simulink model "PR_Planar_Testbench_2018"  (R2024a)
settings: Solver=FixedStepDiscrete  StartTime=0.0  StopTime=inf  FixedStep=param.t_sample  RelTol=1e-3
undefined symbols (not defined in the file): max_qa, min_qa, param, slave3
libraries: Cust_Library_planarPKM x54, simulink_extras x27, dspswit3 x24, simulink x22, etherlab_lib x12
(part 2 of 6)

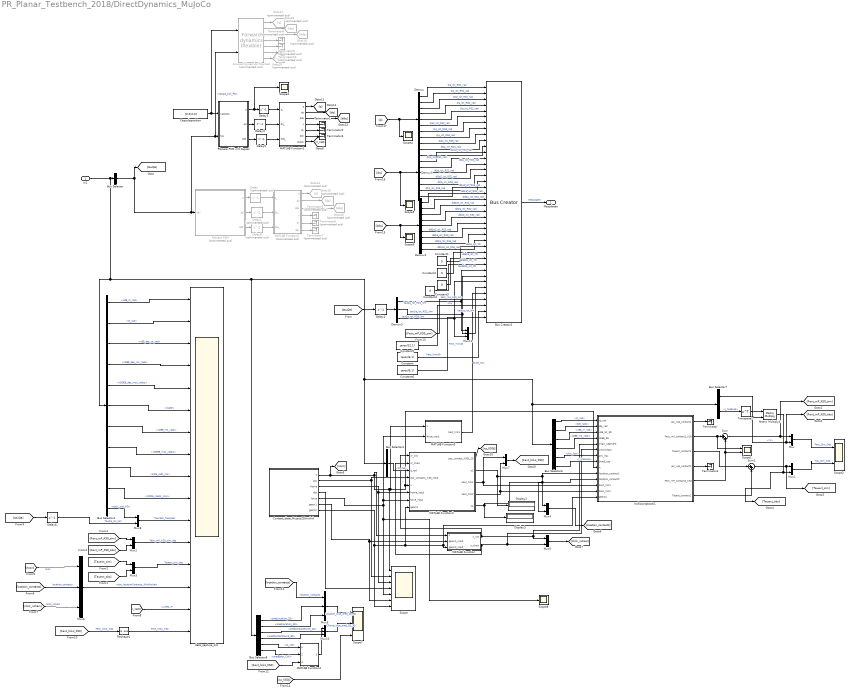
== system PR_Planar_Testbench_2018/DirectDynamics_MuJoCo ==
  In1 : Inport
  Bus Creator2 : BusCreator  Inputs=40
  Bus Selector : BusSelector  OutputSignals=PD_Controller.TauQa_soll_PD
  Bus Selector1 : BusSelector  OutputSignals=Kinematics_currentValues.xEE_m_rad,Kinematics_currentValues.Q_rad,Logical data.xEE_des_m_rad,Logical data.xDEE_des_ms_rads,Logical data.xDDEE_des_mss_radss,Logical data.state,Differential kinematics - current values.xDEE_ms_rads,Differential kinematics - current values.xDDEE_mss_radss,Differential kinematics - current values.QDa_rads_ms,Differential kinematics - current values.QDDa_radss_mss,PD_Controller.tauX_soll_PD
  Bus Selector4 : BusSelector  OutputSignals=Kinematics_currentValues.Q_rad
  Bus Selector6 : BusSelector  OutputSignals=Kinematics_currentValues.Q_rad,Differential kinematics - current values.QD_rads,Kinematics_currentValues.xEE_m_rad,Differential kinematics - current values.xDEE_ms_rads,Differential kinematics - current values.Jinv_hqx,Differential kinematics - current values.J_hredxqa
  Bus Selector7 : BusSelector  OutputSignals=Beobachter.rx,Differential kinematics - current values.J_hredxqa
  Bus Selector8 : BusSelector  OutputSignals=Beobachter.predLocation_2D,Beobachter.predLocation_3D,Beobachter.predContactForce_2D,Beobachter.predContactForce_3D,Kinematics_currentValues.Q_rad,Beobachter.predBody_Coll
  Capsuleposition : Constant  Value=[0;0;0;0]  SampleTime=-1
  Constant : Constant  Value=zeros(6,1)  SampleTime=-1
  Constant{1..4} (4 alike) : Constant  Value=0  SampleTime=-1
  Constant5 : Constant  Value=zeros(12,1)  SampleTime=-1
  Constant6 : Constant  Value=zeros(6,1)  SampleTime=-1
  Contact_data_Mujoco2Simulink : MATLAB Function  TreatAsAtomicUnit=on
  Delay : Delay  Commented=on  DelayLength=1  InitialCondition=param.q0_mj
  Delay1 : Delay  Commented=on  DelayLength=1
  Delay{2,4..6} (4 alike) : Delay  DelayLength=1
  Delay3 : Delay  DelayLength=1  InitialCondition=param.q0_mj
  Delay8 : Delay  Commented=on  DelayLength=1
  Demux : Demux  Outputs=9
  Demux1 : Demux  Outputs=9
  Demux2 : Demux  Outputs=9
  Demux3 : Demux  Outputs=3
  Display2 : Display
  Display3 : Display
  Forward dynamics (flexible) : Cust_Library_planarPKM/Forward dynamics (flexible)  Commented=on  capsule_active=param.capsule_active  t_sample=param.t_sample
  Goto14 : Goto  Commented=on  GotoTag=q
  Goto15 : Goto  Commented=on  GotoTag=dq
  Goto16 : Goto  Commented=on  GotoTag=ddq
  Goto17 : Goto  Commented=on  GotoTag=q
  Goto18 : Goto  Commented=on  GotoTag=dq
  Goto19 : Goto  Commented=on  GotoTag=ddq
  Goto20 : Goto  Commented=on  GotoTag=x_caps
  KollisionsJacobi1 : MATLAB Function  TreatAsAtomicUnit=on
  MATLAB Function : MATLAB Function  TreatAsAtomicUnit=on
  MATLAB Function1 : MATLAB Function  TreatAsAtomicUnit=on
  MATLAB Function2 : MATLAB Function  Commented=on  TreatAsAtomicUnit=on
  MATLAB Function3 : MATLAB Function  TreatAsAtomicUnit=on
  MATLAB Function4 : MATLAB Function  TreatAsAtomicUnit=on
  MATLAB Function5 : MATLAB Function  TreatAsAtomicUnit=on
  Matrix Multiply4 : Product  Multiplication=Matrix(*)
  Mux{,1..5,7..8} (8 alike) : Mux  Inputs=2
  Mux{6,9..11} (4 alike) : Mux  Inputs=3
  Planare PKM : MATLAB Function  Commented=on  TreatAsAtomicUnit=on
  Planare PKM mit Kapsel : MATLAB Function  TreatAsAtomicUnit=on
  Reshape1 : Reshape
  Scope : Scope  NumInputPorts=7
  Scope1 : Scope  NumInputPorts=2
  Scope2 : Scope  NumInputPorts=2
  Scope{3..6,8} (5 alike) : Scope
  Scope7 : Scope  NumInputPorts=3
  Sum : Sum  Inputs=|++
  Sum1 : Sum  Inputs=|++
  Terminator{,1..4} (5 alike) : Terminator
  Terminator{5..10} (6 alike) : Terminator  Commented=on
  Transpose2 : Math  Operator=transpose  SignedPower=on
  data_capture_sim : Scope  NumInputPorts=16
  Messdaten : Outport
  wires:
  Demux/9 -> Bus Creator2/9  "Qp2_ist_RS3_rad"
  Demux1/3 -> Bus Creator2/12  "dQp2_ist_RS1_rad"
  Demux1/8 -> Bus Creator2/17  "dQp_ist_RS3_rad"
  Demux3/3 -> Bus Creator2/34, Mux11/3  "tauQa_ist_RD3_Nm"
  Demux1/1 -> Bus Creator2/10  "dQa_ist_RD1_rad"
  Demux/2 -> Bus Creator2/2  "Qp_ist_RS1_rad"
  Demux/1 -> Bus Creator2/1  "Qa_ist_RD1_rad"
  Demux/4 -> Bus Creator2/4  "Qa_ist_RD2_rad"
  Constant2/1 -> Bus Creator2/29  "ddelta_ist_TD"
  Bus Selector/1 -> [tauQa], Forward dynamics (flexible)/2, Planare PKM mit Kapsel/2(tau), Planare PKM/1(tau)  "<TauQa_soll_PD>"
  Demux/8 -> Bus Creator2/8  "Qp_ist_RS3_rad"
  Delay8/1 -> MATLAB Function2/3(ddq_)
  Demux3/2 -> Mux11/2, Bus Creator2/33  "tauQa_ist_RD2_Nm"
  MATLAB Function2/6(ddx) -> Terminator7/1
  Constant4/1 -> Bus Creator2/31  "taudelta_ist_TD"
  Demux/3 -> Bus Creator2/3  "Qp2_ist_RS1_rad"
  Demux1/7 -> Bus Creator2/16  "dQa_ist_RD3_rad"
  Demux2/5 -> Bus Creator2/23  "ddQp_ist_RS2_rad"
  Demux2/7 -> Bus Creator2/25  "ddQa_ist_RD3_rad"
  Delay2/1 -> Demux3/1
  Demux2/3 -> Bus Creator2/21  "ddQp2_ist_RS1_rad"
  Delay/1 -> MATLAB Function2/1(q_)
  Demux1/9 -> Bus Creator2/18  "dQp2_ist_RS3_rad"
  Demux2/8 -> Bus Creator2/26  "ddQp_ist_RS3_rad"
  Demux2/2 -> Bus Creator2/20  "ddQp_ist_RS1_rad"
  Demux2/4 -> Bus Creator2/22  "ddQa_ist_RD2_rad"
  Demux2/1 -> Bus Creator2/19  "ddQa_ist_RD1_rad"
  Demux1/5 -> Bus Creator2/14  "dQp_ist_RS2_rad"
  Planare PKM/1(q) -> Delay/1
  Demux2/6 -> Bus Creator2/24  "ddQp2_ist_RS2_rad"
  MATLAB Function2/5(dx) -> Terminator6/1
  Demux1/2 -> Bus Creator2/11  "dQp_ist_RS1_rad"
  Demux/5 -> Bus Creator2/5  "Qp_ist_RS2_rad"
  Demux1/4 -> Bus Creator2/13  "dQa_ist_RD2_rad"
  Planare PKM/2(qd) -> Delay1/1
  In1/1 -> Bus Selector8/1, Bus Selector4/1, Bus Selector7/1, Bus Selector6/1, Bus Selector1/1, Bus Selector/1
  Demux2/9 -> Bus Creator2/27  "ddQp2_ist_RS3_rad"
  Demux3/1 -> Mux11/1, Bus Creator2/32  "tauQa_ist_RD1_Nm"
  Constant1/1 -> Bus Creator2/28  "delta_ist_TD"
  Demux1/6 -> Bus Creator2/15  "dQp2_ist_RS2_rad"
  Demux/6 -> Bus Creator2/6  "Qp2_ist_RS2_rad"
  MATLAB Function2/4(x) -> Terminator5/1
  Planare PKM/3(qdd) -> Delay8/1
  Constant3/1 -> Bus Creator2/30  "dddelta_ist_TD"
  Delay1/1 -> MATLAB Function2/2(dq_)
  Demux/7 -> Bus Creator2/7  "Qa_ist_RD3_rad"
  [tauQa] -> Delay2/1
  Bus Creator2/1 -> Messdaten/1  "Messdaten"
  Planare PKM mit Kapsel/1(q) -> Scope3/1, Delay3/1
  Capsuleposition/1 -> Forward dynamics (flexible)/1, Planare PKM mit Kapsel/1(capspos)
  Planare PKM mit Kapsel/3(qdd) -> Delay5/1
  Delay3/1 -> MATLAB Function1/1(q_)
  Delay5/1 -> MATLAB Function1/3(ddq_)
  Delay4/1 -> MATLAB Function1/2(dq_)
  Planare PKM mit Kapsel/2(qd) -> Delay4/1
  MATLAB Function1/4(x) -> Terminator1/1
  MATLAB Function1/5(dx) -> Terminator2/1
  MATLAB Function1/6(ddx) -> Terminator3/1
  Contact_data_Mujoco2Simulink/7(geom2) -> MATLAB Function3/8(geom2), KollisionsJacobi1/14(geom2), MATLAB Function/3(geom2_input), Scope/7
  Contact_data_Mujoco2Simulink/5(force) -> MATLAB Function3/7(force_input), MATLAB Function5/2(force_input), Scope/5, Scope8/1
  Contact_data_Mujoco2Simulink/4(dist) -> Scope/4
  Contact_data_Mujoco2Simulink/3(frame) -> Scope/3, MATLAB Function3/6(frame_input)
  Contact_data_Mujoco2Simulink/2(pos) -> Scope/2, MATLAB Function3/4(pos_contacts_KS0_input)
  Contact_data_Mujoco2Simulink/1(n) -> [ncon], MATLAB Function/1(n), MATLAB Function5/1(n), MATLAB Function3/5(n), KollisionsJacobi1/9(n), Scope/1
  Contact_data_Mujoco2Simulink/6(geom1) -> Scope/6, MATLAB Function/2(geom1_input)
  Bus Selector1/1 -> data_capture_sim/1  "<xEE_m_rad>"
  Bus Selector1/2 -> data_capture_sim/2  "<Q_rad>"
  Bus Selector1/3 -> data_capture_sim/3  "<xEE_des_m_rad>"
  Bus Selector1/4 -> data_capture_sim/4  "<xDEE_des_ms_rads>"
  Bus Selector1/5 -> data_capture_sim/5  "<xDDEE_des_mss_radss>"
  Bus Selector1/6 -> data_capture_sim/6  "<state>"
  Bus Selector1/7 -> data_capture_sim/7  "<xDEE_ms_rads>"
  Bus Selector1/8 -> data_capture_sim/8  "<xDDEE_mss_radss>"
  Bus Selector1/9 -> data_capture_sim/9  "<QDa_rads_ms>"
  Bus Selector1/10 -> data_capture_sim/10  "<QDDa_radss_mss>"
  MATLAB Function3/3(Fext_link1) -> Mux7/1, KollisionsJacobi1/12(Fext_link1)
  MATLAB Function3/4(Fext_link2) -> Mux7/2, KollisionsJacobi1/13(Fext_link2)
  Bus Selector4/1 -> MATLAB Function3/3(q_rad)  "<Q_rad>"
  Bus Selector6/1 -> KollisionsJacobi1/1(qj_rad)  "<Q_rad>"
  Bus Selector6/2 -> KollisionsJacobi1/2(dqj_rad)  "<QD_rads>"
  Bus Selector6/3 -> KollisionsJacobi1/3(xEE_ist_3D)  "<xEE_m_rad>"
  Bus Selector6/4 -> KollisionsJacobi1/4(dxEE_3D)  "<xDEE_ms_rads>"
  Bus Selector6/5 -> KollisionsJacobi1/7(Jinv_hqx)  "<Jinv_hqx>"
  Bus Selector6/6 -> KollisionsJacobi1/8(Jhred_xqa)  "<J_hredxqa>"
  MATLAB Function3/2(s1) -> Display2/1, Mux4/1, KollisionsJacobi1/10(location_contact1)
  MATLAB Function3/5(s2) -> Mux4/2, KollisionsJacobi1/11(location_contact2), Display3/1
  KollisionsJacobi1/1(Jac_xpq_contact1) -> Terminator/1
  KollisionsJacobi1/4(Jac_xpq_contact2) -> Terminator4/1
  KollisionsJacobi1/2(Fext_mP_contact1_KS0) -> Scope1/1, Sum/1
  KollisionsJacobi1/5(Fext_mP_contact2_KS0) -> Scope1/2, Sum/2
  Sum1/1 -> [Tauext_sim], Mux1/1
  KollisionsJacobi1/3(Tauext_contact1) -> Sum1/1
  KollisionsJacobi1/6(Tauext_contact2) -> Sum1/2
  Bus Selector7/1 -> [Fext_mP_KS0_obs], Mux/2, Matrix Multiply4/2  "<rx>"
  Transpose2/1 -> Matrix Multiply4/1
  Bus Selector7/2 -> Transpose2/1  "<J_hredxqa>"
  Matrix Multiply4/1 -> Mux1/2, [Tauext_obs]
  Sum/1 -> [Fext_mP_KS0_sim], Mux/1
  Mux/1 -> Scope2/1  "Fext_Sim_Obs"
  Mux1/1 -> Scope2/2  "Tau_Sim_Obs"
  MATLAB Function/1(n_link) -> MATLAB Function3/1(nr_link), KollisionsJacobi1/5(chain_segment), Mux5/1
  MATLAB Function/2(n_chain) -> KollisionsJacobi1/6(whichchain), Mux5/2, MATLAB Function3/2(nr_chain)
  [Fext_mP_KS0_sim] -> Mux2/1
  [Fext_mP_KS0_obs] -> Mux2/2
  [Tauext_sim] -> Mux3/1
  [Tauext_obs] -> Mux3/2
  Mux2/1 -> data_capture_sim/12  "Fext_mP_KS0_sim_obs"
  Mux3/1 -> data_capture_sim/13  "Tauext_sim_obs"
  Mux4/1 -> [location_contacts]
  Mux5/1 -> [nlink_nchain]
  MATLAB Function1/7(qcaps) -> [x_caps]
  [ncon] -> Mux6/1  "ncon"
  [location_contacts] -> Mux6/2  "location_contacts"
  [nlink_nchain] -> Mux6/3  "nlink_nchain"
  Mux6/1 -> data_capture_sim/14  "ncon_locationContacts_NlinkNchain"
  [x_caps] -> data_capture_sim/15  "x_caps_m"
  [tauQa] -> Delay6/1
  Mux7/1 -> [Fext_links_KS0]
  [Fext_links_KS0] -> Reshape1/1  "Fext_links_KS0"
  Bus Selector1/11 -> Mux8/1  "<tauX_soll_PD>"
  Delay6/1 -> Mux8/2  "TauQa_ist_Nm"
  Mux8/1 -> data_capture_sim/11  "TauXSoll_TauQaIst"
  MATLAB Function1/1(q) -> [q]
  MATLAB Function1/2(dq) -> [dq]
  MATLAB Function1/3(ddq) -> [ddq]
  Bus Selector8/5 -> MATLAB Function4/1(q)  "<Q_rad>"
  Bus Selector8/6 -> MATLAB Function4/2(predBody)  "<predBody_Coll>"
  [Fext_links_KS0] -> MATLAB Function4/3(Fext_links_KS0)
  [location_contacts] -> Mux9/1  "location_contacts"
  Bus Selector8/1 -> Mux9/2  "<predLocation_2D>"
  Bus Selector8/3 -> Mux10/2  "<predContactForce_2D>"
  Mux9/1 -> Scope7/1  "Location_true_pred_2D_3D"
  Mux10/1 -> Scope7/2  "CForce_true_pred_2D_3D"
  MATLAB Function4/1(Fext_link_KSGj) -> Mux10/1
  Bus Selector8/4 -> Mux10/3  "<predContactForce_3D>"
  Bus Selector8/2 -> Mux9/3  "<predLocation_3D>"
  Mux11/1 -> Bus Creator2/35  "tauQa_ist_Nm"
  MATLAB Function5/1(Fext_link1) -> Bus Creator2/36  "force_mjc"
  [Fext_mP_KS0_sim] -> Bus Creator2/37  "Fext_mp_KS0_sim"
  MATLAB Function3/1(pos_contact_KSGj_2D) -> [xp_KSGj]
  [xp_KSGj] -> Scope7/3
  [q] -> Scope4/1, Demux/1
  [dq] -> Scope5/1, Demux1/1
  [ddq] -> Scope6/1, Demux2/1
  MATLAB Function2/2(dq) -> Goto15/1
  MATLAB Function2/3(ddq) -> Goto16/1
  MATLAB Function2/1(q) -> Goto14/1
  Constant5/1 -> Bus Creator2/38  "imu"
  Reshape1/1 -> data_capture_sim/16  "Fext_links_KS0"
  Constant6/1 -> Bus Creator2/40  "Fext_mini40"
  Constant/1 -> Bus Creator2/39  "Fext_kms40"
  Forward dynamics (flexible)/3 -> Goto19/1
  Forward dynamics (flexible)/2 -> Goto18/1
  Forward dynamics (flexible)/1 -> Goto17/1
  Forward dynamics (flexible)/7 -> Goto20/1
  Forward dynamics (flexible)/6 -> Terminator10/1
  Forward dynamics (flexible)/5 -> Terminator9/1
  Forward dynamics (flexible)/4 -> Terminator8/1

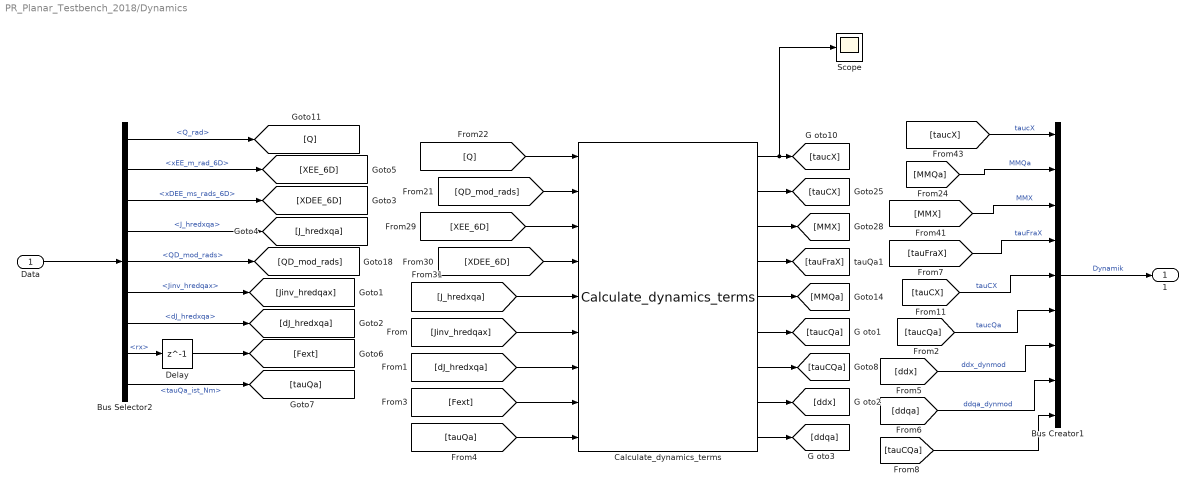
== system PR_Planar_Testbench_2018/Dynamics ==
  Data : Inport
  Bus Creator1 : BusCreator  Inputs=9
  Bus Selector2 : BusSelector  OutputSignals=Kinematics_currentValues.Q_rad,Kinematics_currentValues.xEE_m_rad_6D,Differential kinematics - current values.xDEE_ms_rads_6D,Differential kinematics - current values.J_hredxqa,Differential kinematics - current values.QD_mod_rads,Differential kinematics - current values.Jinv_hredqax,Differential kinematics - current values.dJ_hredxqa,Beobachter.rx,Messdaten.tauQa_ist_Nm
  Calculate_dynamics_terms : Cust_Library_planarPKM/Calculate_dynamics_terms  MDP=param.MDP  l_all=param.l_all  r_BasisPla_MobPla=param.r_BasisPla_MobPla
  Delay : Delay  DelayLength=1  InitialCondition=zeros(3,1)
  Scope : Scope
  1 : Outport
  wires:
  Bus Creator1/1 -> 1/1  "Dynamik"
  [taucX] -> Bus Creator1/1  "taucX"
  [MMX] -> Bus Creator1/3  "MMX"
  [tauFraX] -> Bus Creator1/4  "tauFraX"
  Bus Selector2/3 -> [XDEE_6D]  "<xDEE_ms_rads_6D>"
  Bus Selector2/1 -> [Q]  "<Q_rad>"
  Data/1 -> Bus Selector2/1
  Bus Selector2/4 -> [J_hredxqa]  "<J_hredxqa>"
  Bus Selector2/2 -> [XEE_6D]  "<xEE_m_rad_6D>"
  Bus Selector2/5 -> [QD_mod_rads]  "<QD_mod_rads>"
  [tauCX] -> Bus Creator1/5  "tauCX"
  [MMQa] -> Bus Creator1/2  "MMQa"
  [XEE_6D] -> Calculate_dynamics_terms/3
  [Q] -> Calculate_dynamics_terms/1
  [QD_mod_rads] -> Calculate_dynamics_terms/2
  [XDEE_6D] -> Calculate_dynamics_terms/4
  [J_hredxqa] -> Calculate_dynamics_terms/5
  Calculate_dynamics_terms/1 -> Scope/1, [taucX]
  Calculate_dynamics_terms/2 -> [tauCX]
  Calculate_dynamics_terms/3 -> [MMX]
  Calculate_dynamics_terms/4 -> [tauFraX]
  Calculate_dynamics_terms/5 -> [MMQa]
  Bus Selector2/6 -> [Jinv_hredqax]  "<Jinv_hredqax>"
  [Jinv_hredqax] -> Calculate_dynamics_terms/6
  Bus Selector2/7 -> [dJ_hredxqa]  "<dJ_hredxqa>"
  [dJ_hredxqa] -> Calculate_dynamics_terms/7
  Calculate_dynamics_terms/6 -> [taucQa]
  [taucQa] -> Bus Creator1/6  "taucQa"
  Bus Selector2/8 -> Delay/1  "<rx>"
  [Fext] -> Calculate_dynamics_terms/8
  Bus Selector2/9 -> [tauQa]  "<tauQa_ist_Nm>"
  [tauQa] -> Calculate_dynamics_terms/9
  Calculate_dynamics_terms/8 -> [ddx]
  Calculate_dynamics_terms/9 -> [ddqa]
  Delay/1 -> [Fext]
  [ddx] -> Bus Creator1/7  "ddx_dynmod"
  [ddqa] -> Bus Creator1/8  "ddqa_dynmod"
  Calculate_dynamics_terms/7 -> [tauCQa]
  [tauCQa] -> Bus Creator1/9

== system PR_Planar_Testbench_2018/Init_Block ==
  Start_int : Inport
  Bus Creator : BusCreator  Inputs=5
  Bus Selector : BusSelector  OutputSignals=Statusword.Statusword_RD1,Statusword.Statusword_RD2,Statusword.Statusword_RD3,Statusword.Statusword_TD,Logical data.BP_isError,Controlpanel.Enable_Drive
  Constant : Constant  Value=0  SampleTime=-1
  Constant1 : Constant  SampleTime=-1
  Controlword_Generator : Cust_Library_planarPKM/Controlword_Generator
  Controlword_Generator1 : Cust_Library_planarPKM/Controlword_Generator
  Controlword_Generator2 : Cust_Library_planarPKM/Controlword_Generator
  Controlword_Generator_Translat_Drive : Cust_Library_planarPKM/Controlword_Generator_Translat_Drive
  Data Type Conversion{1..4} (4 alike) : DataTypeConversion  OutDataTypeStr=uint16  SaturateOnIntegerOverflow=off  RndMeth=Floor
  Equal : RelationalOperator  Operator===  OutDataTypeStr=boolean  RndMeth=Simplest  InputSameDT=off
  MATLAB Function : MATLAB Function  TreatAsAtomicUnit=on
  Product{,1..3} (4 alike) : Product
  Switch : Switch  Criteria=u2 > Threshold  SaturateOnIntegerOverflow=off  InputSameDT=off
  Out1 : Outport
  wires:
  Product/1 -> Data Type Conversion3/1
  Controlword_Generator/1 -> Product/1
  [Statusword_RD1] -> Controlword_Generator/1
  Controlword_Generator1/1 -> Product1/1
  Controlword_Generator2/1 -> Product2/1
  [Statusword_RD2] -> Controlword_Generator1/1
  [Statusword_RD3] -> Controlword_Generator2/1
  Product1/1 -> Data Type Conversion1/1
  Product2/1 -> Data Type Conversion2/1
  Data Type Conversion3/1 -> Bus Creator/1, MATLAB Function/1(Controlword_S1)  "Controlword_RD1"
  Data Type Conversion1/1 -> Bus Creator/2, MATLAB Function/2(Controlword_S2)  "Controlword_RD2"
  Data Type Conversion2/1 -> MATLAB Function/3(Controlword_S3), Bus Creator/3  "Controlword_RD3"
  Bus Creator/1 -> Out1/1  "State Variables"
  MATLAB Function/1(Controlword) -> Bus Creator/4  "Controlword"
  Start_int/1 -> Bus Selector/1
  Bus Selector/1 -> [Statusword_RD1]  "<Statusword_RD1>"
  Bus Selector/3 -> [Statusword_RD3]  "<Statusword_RD3>"
  Bus Selector/2 -> [Statusword_RD2]  "<Statusword_RD2>"
  Bus Selector/4 -> [Statusword_TD]  "<Statusword_TD>"
  [Statusword_TD] -> Controlword_Generator_Translat_Drive/1
  Product3/1 -> Data Type Conversion4/1
  Controlword_Generator_Translat_Drive/1 -> Product3/1
  Data Type Conversion4/1 -> Bus Creator/5  "Controlword_TD"
  Constant1/1 -> Equal/2
  Switch/1 -> Controlword_Generator_Translat_Drive/2, Product3/2, Product2/2, Controlword_Generator2/2, Controlword_Generator1/2, Controlword_Generator/2, Product/2, Product1/2
  Constant/1 -> Switch/1
  Bus Selector/5 -> Equal/1  "<BP_isError>"
  Bus Selector/6 -> Switch/3  "<Enable_Drive>"
  Equal/1 -> Switch/2

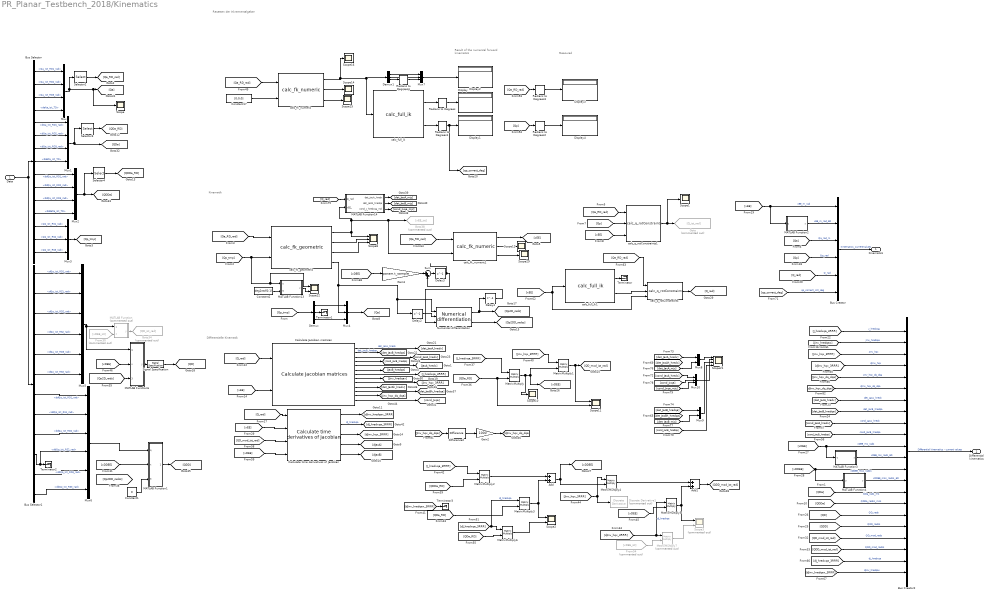
== system PR_Planar_Testbench_2018/Kinematics ==
  note: Resetten der Inkrementalgeber
  note: Kinematik
  note: Measured
  note: Result of the numerical
      | forward kinematics
  note: Differentielle Kinematik
  Data : Inport
  Add : Sum
  Add1 : Sum
  Bus Creator : BusCreator  Inputs=6
  Bus Creator2 : BusCreator  Inputs=22
  Bus Selector : BusSelector  OutputSignals=Messdaten.Qa_ist_RD1_rad,Messdaten.Qa_ist_RD2_rad,Messdaten.Qa_ist_RD3_rad,Messdaten.delta_ist_TD,Messdaten.dQa_ist_RD1_rad,Messdaten.dQa_ist_RD2_rad,Messdaten.dQa_ist_RD3_rad,Messdaten.ddelta_ist_TD,Messdaten.ddQa_ist_RD1_rad,Messdaten.ddQa_ist_RD2_rad,Messdaten.ddQa_ist_RD3_rad,Messdaten.dddelta_ist_TD,Messdaten.Qp_ist_RS1_rad,Messdaten.Qp_ist_RS2_rad,Messdaten.Qp_ist_RS3_rad
  Bus Selector1 : BusSelector  OutputSignals=Messdaten.dQa_ist_RD1_rad,Messdaten.dQp_ist_RS1_rad,Messdaten.dQa_ist_RD2_rad,Messdaten.dQp_ist_RS2_rad,Messdaten.dQa_ist_RD3_rad,Messdaten.dQp_ist_RS3_rad,Messdaten.ddQa_ist_RD1_rad,Messdaten.ddQp_ist_RS1_rad,Messdaten.ddQa_ist_RD2_rad,Messdaten.ddQp_ist_RS2_rad,Messdaten.ddQa_ist_RD3_rad,Messdaten.ddQp_ist_RS3_rad
  Calculate Jacobian matrices : Cust_Library_planarPKM/Calculate Jacobian matrices  l_all_id=param.l_all_id  r_fixPlat_j=param.r_fixPlat_j  r_mobPlat_j=param.r_mobPlat_j  psi_j=param.psi_j  beta_j=param.beta_j
  Calculate time derivatives of Jacobian : Cust_Library_planarPKM/Calculate time derivatives of Jacobian  l_all=param.l_all  r_BasisPla_MobPla=param.r_BasisPla_MobPla
  Constant1 : Constant  Value=0  SampleTime=-1
  Constant17 : Constant  Value=[0;0;0]  SampleTime=-1
  Constant2 : Constant  Value=deg2rad(0.1)  SampleTime=-1
  Delay2 : Delay  DelayLength=1  InitialCondition=param.qp0(2)
  Delay3 : Delay  DelayLength=1  InitialCondition=param.X0_t([1 2 6])
  Delay4 : Delay  DelayLength=1
  Demux : Demux  Outputs=3
  Demux1 : Demux  Outputs=3
  Difference2 : simulink/Discrete/Difference  ICPrevInput=zeros(9,3)  OutMin=[]  OutMax=[]  OutDataType=fixdt(1, 16)  OutScaling=2^-10  DoSatur=off
  Discrete Derivative1 : simulink/Discrete/Discrete Derivative  Commented=on  gainval=1  ICPrevScaledInput=0.0  OutMin=[]  OutMax=[]  OutDataType=fixdt(1, 16)  OutScaling=2^-10  DoSatur=off
  Display{,1..4} (5 alike) : Display
      settings: Decimation=6
  From30 : From  Commented=on  GotoTag=xDEE_ist
  From54 : From  Commented=on  GotoTag=xDEE_ist
  Gain2 : Gain  Gain=1000
  Gain3 : Gain  Gain=param.t_sample
  Goto : Goto  Commented=on  GotoTag=Q_ist_rad
  Goto34 : Goto  Commented=on  GotoTag=QD_ist_rad
  Goto38 : Goto  Commented=on  GotoTag=xEE_ist
  MATLAB Function : MATLAB Function  Commented=on  TreatAsAtomicUnit=on
  MATLAB Function1 : MATLAB Function  TreatAsAtomicUnit=on
  MATLAB Function13 : MATLAB Function  TreatAsAtomicUnit=on
  MATLAB Function14 : MATLAB Function  TreatAsAtomicUnit=on
  MATLAB Function2 : MATLAB Function  TreatAsAtomicUnit=on
  MATLAB Function3 : MATLAB Function  TreatAsAtomicUnit=on
  MATLAB Function4 : MATLAB Function  TreatAsAtomicUnit=on
  MATLAB Function6 : MATLAB Function  TreatAsAtomicUnit=on
  MatrixMultiply{,1..6} (7 alike) : Product  Multiplication=Matrix(*)
  MatrixMultiply7 : Product  Commented=on  Multiplication=Matrix(*)
  Mux : Mux
  Mux1 : Mux
  Mux{3..4,7,10} (4 alike) : Mux  Inputs=3
  Mux2 : Mux
  Mux5 : Mux  Inputs=6
  Mux6 : Mux  Inputs=6
  Mux8 : Mux  Inputs=2
  Mux9 : Mux  Inputs=2
  Numerical differentiation : Cust_Library_planarPKM/Numerical differentiation  t_sample=param.t_sample
  Radians to Degrees{,1..4} (5 alike) : simulink_extras/Transformations/Radians to Degrees
  Scope{,1,10,12,14..16,29} (8 alike) : Scope
  Scope11 : Scope  NumInputPorts=2
  Scope2 : Scope  NumInputPorts=2
  Scope21 : Scope  NumInputPorts=4
  Scope22 : Scope  NumInputPorts=2
  Scope3 : Scope  Commented=on  NumInputPorts=2
  Scope8 : Scope  NumInputPorts=3
  Selector2 : Selector  InputPortWidth=4  IndexOptions=Index vector (dialog)  Indices=[1 2 3]  OutputSizes=1
  Selector3 : Selector  InputPortWidth=4  IndexOptions=Index vector (dialog)  Indices=[1 2 3]  OutputSizes=1
  Selector4 : Selector  InputPortWidth=4  IndexOptions=Index vector (dialog)  Indices=[1 2 3]  OutputSizes=1
  Signal Specification : SignalSpecification  Dimensions=[9 1]
  Sum : Sum  Inputs=|++
  Terminator{,1..3} (4 alike) : Terminator
  calc_fk_geometric : Cust_Library_planarPKM/calc_fk_geometric  psi_j=param.psi_j  beta_j=param.beta_j  r_fixPlat_j=param.r_fixPlat_j  r_mobPlat_j=param.r_mobPlat_j  l_all_id=param.l_all_id
  calc_fk_numeric : Cust_Library_planarPKM/calc_fk_numeric  psi_j=param.psi_j  beta_j=param.beta_j  r_fixPlat_j=param.r_fixPlat_j  r_mobPlat_j=param.r_mobPlat_j  l_all_id=param.l_all_id  max_iter_find_fk_simulink=param.max_iter_find_fk_simulink  max_radius=param.max_radius  max_phie=param.max_phie  min_det_JacA_hredx=param.min_det_JacA_hredx  min_det_JacB_hredqa=param.min_det_JacB_hredqa
  calc_fk_numeric1 : Cust_Library_planarPKM/calc_fk_numeric  psi_j=param.psi_j  beta_j=param.beta_j  r_fixPlat_j=param.r_fixPlat_j  r_mobPlat_j=param.r_mobPlat_j  l_all_id=param.l_all_id  max_iter_find_fk_simulink=param.max_iter_find_fk_simulink  max_radius=param.max_radius  max_phie=param.max_phie  min_det_JacA_hredx=param.min_det_JacA_hredx  min_det_JacB_hredqa=param.min_det_JacB_hredqa
  calc_full_ik : Cust_Library_planarPKM/calc_full_ik  psi_j=param.psi_j  beta_j=param.beta_j  r_fixPlat_j=param.r_fixPlat_j  r_mobPlat_j=param.r_mobPlat_j  l_all_id=param.l_all_id
  calc_full_ik1 : Cust_Library_planarPKM/calc_full_ik  psi_j=param.psi_j  beta_j=param.beta_j  r_fixPlat_j=param.r_fixPlat_j  r_mobPlat_j=param.r_mobPlat_j  l_all_id=param.l_all_id
  calc_q_rotConstraints : Cust_Library_planarPKM/calc_q_rotConstraints  psi_j=param.psi_j
  calc_q_rotConstraints1 : Cust_Library_planarPKM/calc_q_rotConstraints  psi_j=param.psi_j
  Kinematics : Outport
  Differential kinematics : Outport  Port=2
  wires:
  Bus Creator/1 -> Kinematics/1  "Kinematics_currentValues"
  Bus Creator2/1 -> Differential kinematics/1  "Differential kinematics - current values"
  [J_hredxqa_3RRR] -> Bus Creator2/1  "J_hredxqa"
  [xDDEE] -> MATLAB Function4/1(u), Bus Creator2/13  "xDDEE_mss_radss"
  Data/1 -> Bus Selector1/1, Bus Selector/1
  Bus Selector/1 -> Mux/1  "<Qa_ist_RD1_rad>"
  Bus Selector/2 -> Mux/2  "<Qa_ist_RD2_rad>"
  Bus Selector/3 -> Mux/3  "<Qa_ist_RD3_rad>"
  Bus Selector/4 -> Mux/4  "<delta_ist_TD>"
  [QDa] -> Bus Creator2/15  "QDa_rads_ms"
  [QDDa] -> Bus Creator2/16  "QDDa_radss_mss"
  [QD] -> Bus Creator2/17  "QD_rads"
  [QDD] -> Bus Creator2/18  "QDD_radss"
  Bus Selector/5 -> Mux1/1  "<dQa_ist_RD1_rad>"
  Bus Selector/6 -> Mux1/2  "<dQa_ist_RD2_rad>"
  Bus Selector/7 -> Mux1/3  "<dQa_ist_RD3_rad>"
  Bus Selector/8 -> Mux1/4  "<ddelta_ist_TD>"
  Bus Selector/9 -> Mux2/1  "<ddQa_ist_RD1_rad>"
  Bus Selector/10 -> Mux2/2  "<ddQa_ist_RD2_rad>"
  Bus Selector/11 -> Mux2/3  "<ddQa_ist_RD3_rad>"
  Mux3/1 -> [Qp_tmp]
  Bus Selector/13 -> Mux3/1  "<Qp_ist_RS1_rad>"
  Bus Selector/14 -> Mux3/2  "<Qp_ist_RS2_rad>"
  Bus Selector/15 -> Mux3/3  "<Qp_ist_RS3_rad>"
  [Qa_RD_rad] -> calc_fk_geometric/1
  calc_fk_geometric/3 -> Scope8/3
  calc_fk_geometric/2 -> Scope8/2
  [Qp_tmp] -> Demux/1
  Demux/1 -> Mux4/1
  Demux/3 -> Mux4/3
  Demux/2 -> Terminator1/1
  Mux4/1 -> [Qp]
  [Qa_RD_rad] -> calc_q_rotConstraints1/1
  [xEE] -> calc_q_rotConstraints1/3
  [Qp] -> calc_q_rotConstraints1/2
  calc_q_rotConstraints1/1 -> Goto/1, Scope1/1
  [Q_rad] -> Calculate Jacobian matrices/1
  Calculate Jacobian matrices/1 -> [det_JacA_hredx]  "det_JacA_hredx"
  Calculate Jacobian matrices/2 -> [det_JacB_hredqa]  "det_JacB_hredqa"
  MatrixMultiply4/1 -> Add1/1
  [J_hredxqa_3RRR] -> MatrixMultiply2/1
  [dJ_hredxqa_3RRR] -> MatrixMultiply3/1, MatrixMultiply6/1  "dJ_hredxqa"
  [QDa_RD] -> MatrixMultiply6/2
  From54/1 -> MatrixMultiply7/2
  [Jinv_hqx_3RRR] -> MatrixMultiply1/1
  [QDa_RD] -> Scope11/2, MatrixMultiply/2
  [J_hredxqa_3RRR] -> MatrixMultiply/1
  MatrixMultiply5/1 -> Scope3/1, Add1/2
  MatrixMultiply1/1 -> Scope11/1, [QD_mod_ist_rad]
  MatrixMultiply7/1 -> Scope3/2
  MatrixMultiply6/1 -> Scope2/2
  Add1/1 -> [QDD_mod_ist_rad]
  Add/1 -> MatrixMultiply4/2, [xDDEE]
  [xDEE] -> MatrixMultiply5/2
  MatrixMultiply2/1 -> Add/1
  [Jinv_hqx_3RRR] -> MatrixMultiply4/1, Discrete Derivative1/1
  MatrixMultiply3/1 -> Add/2, Scope2/1
  [dJinv_hqx_3RRR] -> MatrixMultiply5/1, MatrixMultiply7/1  "dJ_hredxqa"
  [QDa_RD] -> MatrixMultiply3/2
  MatrixMultiply/1 -> Scope10/1, MatrixMultiply1/2, [xDEE]
  [QDDa_RD] -> MatrixMultiply2/2
  Selector2/1 -> [Qa_RD_rad]
  Mux/1 -> Scope/1, [Qa], Selector2/1
  Selector3/1 -> [QDa_RD]
  Mux1/1 -> [QDa], Selector3/1
  Bus Selector/12 -> Mux2/4  "<dddelta_ist_TD>"
  Selector4/1 -> [QDDa_RD]
  Mux2/1 -> [QDDa], Selector4/1
  [xEE] -> MATLAB Function2/1(u), Bus Creator/1  "xEE_m_rad"
  [Qa] -> Bus Creator/3  "Qa_rad_m"
  [Qp] -> Bus Creator/4  "Qp_rad"
  [Q_rad] -> Bus Creator/5  "Q_rad"
  [det_JacB_hredqa] -> Bus Creator2/8  "det_JacB_hredqa"
  [det_JacA_hredx] -> Bus Creator2/7  "det_JacA_hredx"
  [xDEE] -> Bus Creator2/11, MATLAB Function3/1(u)  "xDEE_ms_rads"
  [Jinv_hqx_3RRR] -> Bus Creator2/3  "Jinv_hqx"
  Bus Selector1/1 -> Mux5/1  "<dQa_ist_RD1_rad>"
  Bus Selector1/2 -> Mux5/2  "<dQp_ist_RS1_rad>"
  Bus Selector1/7 -> Mux6/1  "<ddQa_ist_RD1_rad>"
  Bus Selector1/8 -> Mux6/2  "<ddQp_ist_RS1_rad>"
  Bus Selector1/12 -> Mux6/6  "<ddQp_ist_RS3_rad>"
  Bus Selector1/11 -> Mux6/5  "<ddQa_ist_RD3_rad>"
  Bus Selector1/9 -> Mux6/3  "<ddQa_ist_RD2_rad>"
  Bus Selector1/6 -> Mux5/6  "<dQp_ist_RS3_rad>"
  Bus Selector1/5 -> Mux5/5  "<dQa_ist_RD3_rad>"
  Bus Selector1/3 -> Mux5/3  "<dQa_ist_RD2_rad>"
  Mux5/1 -> MATLAB Function/1(q), MATLAB Function6/1(q)
  From30/1 -> MATLAB Function/2(x)
  MATLAB Function/1(y) -> Goto34/1
  [xDDEE] -> MATLAB Function1/2(x)
  Mux6/1 -> MATLAB Function1/1(q)
  MATLAB Function1/1(y_final) -> [QDD]
  MATLAB Function2/1(y) -> Bus Creator/2  "xEE_m_rad_6D"
  MATLAB Function3/1(y) -> Bus Creator2/12  "xDEE_ms_rads_6D"
  MATLAB Function4/1(y) -> Bus Creator2/14  "xDDEE_mss_radss_6D"
  [QD_mod_ist_rad] -> Bus Creator2/19  "QD_mod_rads"
  [QDD_mod_ist_rad] -> Bus Creator2/20  "QDD_mod_radss"
  Delay4/1 -> Numerical differentiation/3
  Numerical differentiation/1 -> [Qp2D_rads], Delay4/1
  calc_fk_geometric/4 -> Numerical differentiation/1, Delay2/1, Mux4/2
  Delay2/1 -> Numerical differentiation/2
  Bus Selector1/4 -> Mux5/4  "<dQp_ist_RS2_rad>"
  Bus Selector1/10 -> Mux6/4, Terminator2/1  "<ddQp_ist_RS2_rad>"
  [dJinv_hredqax_3RRR] -> Terminator3/1
  Numerical differentiation/2 -> [Qp2DD_radss]
  [xDEE] -> MATLAB Function6/2(x)
  [Qp2D_rads] -> MATLAB Function6/3(qp2D_correct)
  Constant1/1 -> MATLAB Function1/3(qp2DD_correct)
  Calculate time derivatives of Jacobian/3 -> [dJinv_hqx_3RRR]
  [Q_rad] -> Calculate time derivatives of Jacobian/1
  [xDEE] -> Calculate time derivatives of Jacobian/4
  [xEE] -> Calculate time derivatives of Jacobian/2
  Calculate time derivatives of Jacobian/1 -> [dJinv_hredqax_3RRR]
  [QD_mod_ist_rad] -> Calculate time derivatives of Jacobian/3
  Calculate time derivatives of Jacobian/2 -> [dJ_hredxqa_3RRR]  "dJ_hredxqa"
  [dJinv_hqx_3RRR] -> Bus Creator2/4  "dJinv_hqx"
  [Jinv_hredqax] -> Bus Creator2/2  "Jinv_hredqax"
  MATLAB Function6/1(y) -> Signal Specification/1
  Signal Specification/1 -> [QD]
  [Qa_RD_rad] -> calc_fk_numeric1/1
  calc_fk_numeric1/2 -> Scope12/1
  [dJ_hredxqa_3RRR] -> Bus Creator2/21  "dJ_hredxqa"
  [dJinv_hredqax_3RRR] -> Bus Creator2/22  "dJinv_hredqax"
  calc_fk_numeric1/3 -> Scope29/1
  Calculate Jacobian matrices/8 -> [Jinv_hredqax]
  Calculate Jacobian matrices/7 -> [J_hredxqa_3RRR]
  Calculate Jacobian matrices/9 -> [Jinv_hqx_3RRR]
  calc_fk_geometric/1 -> MATLAB Function14/2(xEE_), calc_fk_numeric1/2, Goto38/1, Scope8/1
  calc_fk_numeric1/1 -> [xEE]
  Constant17/1 -> calc_fk_numeric/2
  calc_fk_numeric/3 -> Scope15/1
  calc_fk_numeric/2 -> Scope14/1
  [Qa_RD_rad] -> calc_fk_numeric/1
  calc_fk_numeric/1 -> Scope16/1, calc_full_ik/1, Demux1/1
  calc_full_ik/1 -> Radians to Degrees/1
  calc_full_ik/2 -> Radians to Degrees1/1
  Radians to Degrees1/1 -> [qp_correct_deg], Display1/1
  [qp_correct_deg] -> Bus Creator/6  "qp_correct_init_deg"
  [Qa_RD_rad] -> Radians to Degrees3/1
  Radians to Degrees2/1 -> Display4/1
  [Qp] -> Radians to Degrees2/1
  Radians to Degrees3/1 -> Display3/1
  Radians to Degrees/1 -> Display/1
  Demux1/1 -> Mux7/1
  Mux7/1 -> Display2/1
  Demux1/2 -> Mux7/2
  Demux1/3 -> Radians to Degrees4/1
  Radians to Degrees4/1 -> Mux7/3
  Calculate Jacobian matrices/5 -> [JacA_hredx]
  Calculate Jacobian matrices/6 -> [JacB_hredqa]
  Calculate time derivatives of Jacobian/4 -> [dJacA]
  Calculate time derivatives of Jacobian/5 -> [dJacB]
  Calculate Jacobian matrices/3 -> [cond_JacA_hredx]
  Calculate Jacobian matrices/4 -> [cond_JacB_hredqa]
  [cond_JacB_hredqa] -> Bus Creator2/10  "cond_JacB_hredqa"
  [cond_JacA_hredx] -> Bus Creator2/9  "cond_JacA_hredx"
  [xEE] -> calc_q_rotConstraints/3, calc_full_ik1/1
  calc_full_ik1/2 -> calc_q_rotConstraints/2
  [Qa_RD_rad] -> calc_q_rotConstraints/1
  calc_q_rotConstraints/1 -> [Q_rad]
  Sum/1 -> Delay3/1
  Gain3/1 -> Sum/1
  Delay3/1 -> Sum/2
  [xDEE] -> Gain3/1
  Calculate Jacobian matrices/10 -> [det_JacAh_hredx]
  Calculate Jacobian matrices/11 -> [det_JacBh_hredqa]
  [det_JacB_hredqa] -> Mux9/1
  [det_JacA_hredx] -> Mux8/1
  Mux8/1 -> Scope21/1
  Mux9/1 -> Scope21/3
  [cond_JacB_hredqa] -> Scope21/4
  Constant2/1 -> MATLAB Function13/2(N)
  MATLAB Function13/1(y) -> Scope22/2
  [Qp_tmp] -> calc_fk_geometric/2, MATLAB Function13/1(u), Scope22/1
  [Q_rad] -> MATLAB Function14/1(qj_rad)
  MATLAB Function14/1(det_JacA_hredx) -> [det_JacA_mjc]
  MATLAB Function14/2(det_JacB_hredqa) -> [det_JacB_mjc]
  [det_JacB_mjc] -> Mux9/2
  [det_JacA_mjc] -> Mux8/2
  Calculate Jacobian matrices/13 -> [cond_Jxqa]
  MATLAB Function14/3(cond_J_hredxqa_ind) -> [cond_Jxqa_mjc]
  [cond_JacA_hredx] -> Mux10/1
  [cond_Jxqa] -> Mux10/2
  [cond_Jxqa_mjc] -> Mux10/3
  Mux10/1 -> Scope21/2
  Calculate Jacobian matrices/12 -> [Jinv_hqx_dq_dqa]
  [Jinv_hqx_dq_dqa] -> Bus Creator2/5  "Jinv_hqx_dq_dqa"
  Gain2/1 -> [dJinv_hqx_dq_dqa]
  Difference2/1 -> Gain2/1
  [Jinv_hqx_dq_dqa] -> Difference2/1
  [dJinv_hqx_dq_dqa] -> Bus Creator2/6  "dJinv_hqx_dq_dqa"
  calc_full_ik1/1 -> Terminator/1
  [xEE] -> Calculate Jacobian matrices/2
